simulink model "Scenario_3_PF"  (R2020b)
settings: Solver=ode1  StartTime=0.0  StopTime=10.0  RelTol=1e-3
InitFcn:
  | Scenario_3_parameters;
values from neighbouring files (symbols this model uses):
  c0 = c0_zeb    (= 6.57988e-09)    [Scenario_17_parameters_v2.m]    (also in Scenario_1_parameters_v2.m; Scenario_2_parameters_v2.m; Scenario_3_parameters_v2.m)
  c0_hawk = 6.37282e-09    [Scenario_17_parameters_v2.m]    (also in Scenario_1_parameters_v2.m; Scenario_2_parameters_v2.m; Scenario_3_parameters_v2.m)
  c1 = c1_zeb    (= 9.15905e-09)    [Scenario_17_parameters_v2.m]    (also in Scenario_1_parameters_v2.m; Scenario_2_parameters_v2.m; Scenario_3_parameters_v2.m)
  c1_hawk = 8.76156e-09    [Scenario_17_parameters_v2.m]    (also in Scenario_1_parameters_v2.m; Scenario_2_parameters_v2.m; Scenario_3_parameters_v2.m)
  fg = 50    [Scenario_17_parameters_v2.m]    (also in Scenario_1_parameters_v2.m; Scenario_2_parameters_v2.m; Scenario_3_parameters_v2.m)
  G10gen = 0.90    (= 0.9)    [Scenario_3_parameters_v2.m]
  G12gen = 0.85    [Scenario_3_parameters_v2.m]
  G1gen = 0.4692    [Scenario_17_parameters_v2.m]    (also in Scenario_1_parameters_v2.m = 0.1; Scenario_2_parameters_v2.m = 0.298581; Scenario_3_parameters_v2.m = 0.65)
  G2gen = 0.80    (= 0.8)    [Scenario_1_parameters_v2.m]    (also in Scenario_2_parameters_v2.m = 0.7; Scenario_3_parameters_v2.m = 0.4)
  G3gen = 0.85    [Scenario_1_parameters_v2.m]    (also in Scenario_2_parameters_v2.m = 0.9; Scenario_3_parameters_v2.m = 0.6)
  G4gen = 0.65    [Scenario_3_parameters_v2.m]
  G5gen = 0.75    [Scenario_17_parameters_v2.m]    (also in Scenario_1_parameters_v2.m = 0.8; Scenario_2_parameters_v2.m = 0.8; Scenario_3_parameters_v2.m = 0.705)
  G6gen = 0.90    (= 0.9)    [Scenario_17_parameters_v2.m]    (also in Scenario_1_parameters_v2.m; Scenario_2_parameters_v2.m = 0.81797; Scenario_3_parameters_v2.m = 0.45)
  G7gen = 0.20    (= 0.2)    [Scenario_17_parameters_v2.m]    (also in Scenario_1_parameters_v2.m = 0.5227; Scenario_2_parameters_v2.m = 0.5098; Scenario_3_parameters_v2.m = 0.4)
  G8gen = 0.58    [Scenario_17_parameters_v2.m]    (also in Scenario_3_parameters_v2.m = 0.65)
  G9gen = 0.8833    [Scenario_17_parameters_v2.m]    (also in Scenario_3_parameters_v2.m = 0.9)
  Ihvpk = Ihv*sqrt(2)    [Scenario_17_parameters_v2.m]    (also in Scenario_1_parameters_v2.m; Scenario_2_parameters_v2.m; Scenario_3_parameters_v2.m)
  l0 = l0_zeb    (= 0.00368)    [Scenario_17_parameters_v2.m]    (also in Scenario_1_parameters_v2.m; Scenario_2_parameters_v2.m; Scenario_3_parameters_v2.m)
  l0_hawk = 0.00373    [Scenario_17_parameters_v2.m]    (also in Scenario_1_parameters_v2.m; Scenario_2_parameters_v2.m; Scenario_3_parameters_v2.m)
  l1 = l1_zeb    (= 0.00128)    [Scenario_17_parameters_v2.m]    (also in Scenario_1_parameters_v2.m; Scenario_2_parameters_v2.m; Scenario_3_parameters_v2.m)
  L10dem = 0.04    [Scenario_3_parameters_v2.m]
  L12dem = 0.01    [Scenario_17_parameters_v2.m]    (also in Scenario_3_parameters_v2.m = 0.02)
  L13dem = 0.01    [Scenario_3_parameters_v2.m]
  l1_hawk = 0.00133    [Scenario_17_parameters_v2.m]    (also in Scenario_1_parameters_v2.m; Scenario_2_parameters_v2.m; Scenario_3_parameters_v2.m)
  L1dem = 0.25    [Scenario_17_parameters_v2.m]    (also in Scenario_3_parameters_v2.m = 0.1)
  L3dem = 0.30    (= 0.3)    [Scenario_17_parameters_v2.m]    (also in Scenario_1_parameters_v2.m = 0.1; Scenario_2_parameters_v2.m = 0.1; Scenario_3_parameters_v2.m = 0.2)
  L6dem = 0.15    [Scenario_1_parameters_v2.m]    (also in Scenario_2_parameters_v2.m; Scenario_3_parameters_v2.m = 0.1)
  L7dem = 0.10    (= 0.1)    [Scenario_1_parameters_v2.m]    (also in Scenario_2_parameters_v2.m; Scenario_3_parameters_v2.m = 0.2)
  L9dem = 0.15    [Scenario_17_parameters_v2.m]    (also in Scenario_3_parameters_v2.m = 0.1)
  Pr = Sr*PF    (= 1600500000)    [Scenario_17_parameters_v2.m]    (also in Scenario_1_parameters_v2.m = 1472500000; Scenario_2_parameters_v2.m = 1805000000; Scenario_3_parameters_v2.m = 12740000000)
  Qr = sqrt(Sr^2 - Pr^2)    [Scenario_17_parameters_v2.m]    (also in Scenario_1_parameters_v2.m; Scenario_2_parameters_v2.m; Scenario_3_parameters_v2.m)
  r0 = r0_zeb    (= 0.39362)    [Scenario_17_parameters_v2.m]    (also in Scenario_1_parameters_v2.m; Scenario_2_parameters_v2.m; Scenario_3_parameters_v2.m)
  r0_hawk = 0.44587    [Scenario_17_parameters_v2.m]    (also in Scenario_1_parameters_v2.m; Scenario_2_parameters_v2.m; Scenario_3_parameters_v2.m)
  r1 = r1_zeb    (= 0.06862)    [Scenario_17_parameters_v2.m]    (also in Scenario_1_parameters_v2.m; Scenario_2_parameters_v2.m; Scenario_3_parameters_v2.m)
  r1_hawk = 0.12087    [Scenario_17_parameters_v2.m]    (also in Scenario_1_parameters_v2.m; Scenario_2_parameters_v2.m; Scenario_3_parameters_v2.m)
  Rtpu = Xtpu/40    (= 0.0025)    [Scenario_17_parameters_v2.m]    (also in Scenario_1_parameters_v2.m = 0.00375; Scenario_2_parameters_v2.m = 0.00375; Scenario_3_parameters_v2.m)
  S10non = 500e6    (= 500000000)    [Scenario_3_parameters_v2.m]
  S12non = 250e6    (= 250000000)    [Scenario_3_parameters_v2.m]
  S1non = 700e6    (= 700000000)    [Scenario_17_parameters_v2.m]    (also in Scenario_1_parameters_v2.m = 400000000; Scenario_2_parameters_v2.m = 400000000; Scenario_3_parameters_v2.m = 1000000000)
  S2non = 300e6    (= 300000000)    [Scenario_1_parameters_v2.m]    (also in Scenario_2_parameters_v2.m; Scenario_3_parameters_v2.m = 3000000000)
  S3non = 200e6    (= 200000000)    [Scenario_1_parameters_v2.m]    (also in Scenario_2_parameters_v2.m; Scenario_3_parameters_v2.m = 1000000000)
  S4non = 2000e6    (= 2000000000)    [Scenario_3_parameters_v2.m]
  S5non = 400e6    (= 400000000)    [Scenario_17_parameters_v2.m]    (also in Scenario_1_parameters_v2.m = 500000000; Scenario_2_parameters_v2.m = 500000000; Scenario_3_parameters_v2.m = 2000000000)
  S6non = 150e6    (= 150000000)    [Scenario_17_parameters_v2.m]    (also in Scenario_1_parameters_v2.m = 400000000; Scenario_2_parameters_v2.m = 400000000; Scenario_3_parameters_v2.m = 3000000000)
  S7non = 1500e6    (= 1500000000)    [Scenario_17_parameters_v2.m]    (also in Scenario_1_parameters_v2.m = 200000000; Scenario_2_parameters_v2.m = 200000000; Scenario_3_parameters_v2.m = 4000000000)
  S8non = 600e6    (= 600000000)    [Scenario_17_parameters_v2.m]    (also in Scenario_3_parameters_v2.m = 2000000000)
  S9non = 200e6    (= 200000000)    [Scenario_17_parameters_v2.m]    (also in Scenario_3_parameters_v2.m = 1500000000)
  tonvsc = 0    [Scenario_17_parameters_v2.m]    (also in Scenario_1_parameters_v2.m; Scenario_2_parameters_v2.m; Scenario_3_parameters_v2.m = 0.0001)
  Ts = 50e-6    (= 5e-05)    [Scenario_17_parameters_v2.m]    (also in Scenario_1_parameters_v2.m = 0.0002; Scenario_2_parameters_v2.m = 2e-05; Scenario_3_parameters_v2.m = 0.0001)
  Vhv = 220e3    (= 220000)    [Scenario_17_parameters_v2.m]    (also in Scenario_1_parameters_v2.m; Scenario_2_parameters_v2.m; Scenario_3_parameters_v2.m)
  Vmv = 22e3    (= 22000)    [Scenario_17_parameters_v2.m]    (also in Scenario_1_parameters_v2.m; Scenario_2_parameters_v2.m; Scenario_3_parameters_v2.m)
  wc1 = wsw1/10    (= 848.230016469)    [Scenario_17_parameters_v2.m]    (also in Scenario_1_parameters_v2.m; Scenario_2_parameters_v2.m; Scenario_3_parameters_v2.m)
  wdc1 = wc1/10    (= 84.8230016469)    [Scenario_17_parameters_v2.m]    (also in Scenario_1_parameters_v2.m; Scenario_2_parameters_v2.m; Scenario_3_parameters_v2.m)
  wpq1 = wc1/10    (= 84.8230016469)    [Scenario_17_parameters_v2.m]    (also in Scenario_1_parameters_v2.m; Scenario_2_parameters_v2.m; Scenario_3_parameters_v2.m)
  wsw1 = ksw1*2*pi*fg    (= 8482.30016469)    [Scenario_17_parameters_v2.m]    (also in Scenario_1_parameters_v2.m; Scenario_2_parameters_v2.m; Scenario_3_parameters_v2.m)
  Xtpu = 0.10    (= 0.1)    [Scenario_17_parameters_v2.m]    (also in Scenario_1_parameters_v2.m = 0.15; Scenario_2_parameters_v2.m = 0.15; Scenario_3_parameters_v2.m)
undefined symbols (not defined in the file or in its folder): D11, Delta, Kf, r, theta0
libraries: powerlib x426, simulink_extras x305, powerlib_meascontrol x139, pid_lib x109, eeGeneralControl x72, simulink x60, eeTransforms x54, spsFirstOrderFilterLib x36, eePwmGeneratorTwoLevel x9
(part 5 of 36)

== system Scenario_3_PF/G9 ==
  Bus Selector : BusSelector  OutputSignals=Pabc,Qabc,f
  VSC : Subsystem  mask{vscmod=Phasor I-ref, fg=fg, Vhv=Vmv, Vmv=Vmv, Pconv=S9non, Rtpu=Rtpu, Xtpu=Xtpu, Hvsc=30e-3, qmode=Active power, dmode=Reactive power, wsw=wsw1, wn_pll=2*pi*80, wc=wc1, wpq=wpq1, wdc=wdc1, koc=1.2, tfilt=1*(1/wsw1), negseq_en=off, fdroop_en=on, Vacdroop_en=on, LVRT_en=off, Kfdroop=0.05, Kvdroop=0.1, Vlvrt0=0.9, Vlvrt_min=0.5, Qmax_lvrt=0.9}
      mask prompts: vscmod "VSC Model"; fg "AC grid frequency (Hz)"; Vhv "Grid-side voltage (V)(LL-rms)"; Vmv "Converter-side voltage (V)(LL-rms)"; Pconv "Converter nominal power (VA)"; Rtpu "Resistance seen by the converter (p.u)"; Xtpu "Reactance seen by the converter (p.u)"; Hvsc "VSC equivalent inertia (s)"; qmode "q-axis control mode"; dmode "d-axis control mode"; wsw "Switching frequency (rad/s)"; wn_pll "PLL filter natural frequency"; wc "Current-control bandwidth (rad/s)"; wpq "PQ control bandwidth (rad/s)"; wdc "DC Voltage control bandwidth(rad/s)"; koc "Overcurrent factor (p.u)"; tfilt "Vabc filter time constant (s)"; negseq_en "Enable negative sequence control"; fdroop_en "Enable frequency droop"; Vacdroop_en "Enable AC voltage droop"; LVRT_en "Enable LVRT"; Kfdroop "Frequency droop (p.u)"; Kvdroop "Voltage droop (p.u)"; Vlvrt0 "initial voltage (p.u)"; Vlvrt_min "minimum voltage (p.u)"; Qmax_lvrt "max power injected at min voltage (p.u)"
      mask init: same as Scenario_3_PF/G1/VSC
      mask TypeOptions vscmod: EMT Switching | EMT Average | Phasor Quasi-EMT | Phasor I-1st | Phasor I-ref | Phasor PQ-1st
      mask Callback vscmod:
      | % Control parameter visiblity
      | 
      | % Get the value of the Enable Bias checkbox
      | % unchecked = 'off'
      | % checked = 'on'
      | 
      | maskObj = Simulink.Mask.get(gcb);
      | 
      | wn_pll = 'on';
      | wsw = 'on';
      | vscmod = get_param(gcb,'vscmod');
      |     if strcmp(vscmod,'EMT Switching')
      |       wn_pll = 'on';
      |       wsw = 'on';
      |       tfilt = 'on';
      |     elseif strcmp(vscmod,'EMT Average')
      |         wn_pll = 'on';
      |         wsw = 'off';
      |         tfilt = 'off';
      |     elseif strcmp(vscmod,'Phasor Quasi-EMT')
      |         wn_pll = 'off';
      |         wsw = 'off';
      |         tfilt = 'off';
      |     elseif strcmp(vscmod,'Phasor I-1st')
      |         wn_pll = 'off';
      |         wsw = 'off';
      |         tfilt = 'off';
      |     elseif strcmp(vscmod,'Phasor I-ref')
      |         wn_pll = 'off';
      |         wsw = 'off';
      |         tfilt = 'off';
      |     elseif strcmp(vscmod,'Phasor PQ-1st')
      |         wn_pll = 'off';
      |         wsw = 'off';
      |         tfilt = 'off';
      |     end
      | 
      | fdroop_en = get_param(gcb,'fdroop_en');
      | Vacdroop_en = get_param(gcb,'Vacdroop_en');
      | LVRT_en = get_param(gcb,'LVRT_en');
      | negseq_en = get_param(gcb,'negseq_en');
      | 
      | % Set the 'MaskVisibilities' property for each parameters
      |     set_param(gcb,'MaskVisibilities',{'on','on','on','on','on','on','on','on','on','on',wsw,wn_pll,'on','on','on','on',tfilt,'on','on','on','on',fdroop_en,Vacdroop_en,'on','on','on'});
      | 
      | % Make LVRT area visible when it is enabled
      | if strcmp(LVRT_en,'on')
      |   maskObj.getDialogControl('Container_LVRT').Visible = 'on';
      | else
      |     maskObj.getDialogControl('Container_LVRT').Visible = 'off';
      | end
      | 
      | % Note that the value of the bias is not handled here.
      | % See the Initialization tab
      mask TypeOptions qmode: Active power | DC voltage
      mask Callback qmode:
      | %if strcmp(qmode,'Active Power')
      | %    disp(qmode)
      | %elseif strcmp(qmode,'DC Voltage')
      | %    disp(qmode)
      | %end
      mask TypeOptions dmode: Reactive power | AC voltage
      mask Callback fdroop_en:
      | % Control parameter visiblity
      | 
      | % Get the value of the Enable Bias checkbox
      | % unchecked = 'off'
      | % checked = 'on'
      | 
      | maskObj = Simulink.Mask.get(gcb);
      | 
      | wn_pll = 'on';
      | wsw = 'on';
      | vscmod = get_param(gcb,'vscmod');
      |     if strcmp(vscmod,'EMT Switching')
      |       wn_pll = 'on';
      |       wsw = 'on';
      |       tfilt = 'on';
      |     elseif strcmp(vscmod,'EMT Average')
      |         wn_pll = 'on';
      |         wsw = 'off';
      |         tfilt = 'off';
      |     elseif strcmp(vscmod,'Phasor Quasi-EMT')
      |         wn_pll = 'off';
      |         wsw = 'off';
      |         tfilt = 'off';
      |     elseif strcmp(vscmod,'Phasor I-1st')
      |         wn_pll = 'off';
      |         wsw = 'off';
      |         tfilt = 'off';
      |     elseif strcmp(vscmod,'Phasor I-ref')
      |         wn_pll = 'off';
      |         wsw = 'off';
      |         tfilt = 'off';
      |     elseif strcmp(vscmod,'Phasor PQ-1st')
      |         wn_pll = 'off';
      |         wsw = 'off';
      |         tfilt = 'off';
      |     end
      | 
      | fdroop_en = get_param(gcb,'fdroop_en');
      | Vacdroop_en = get_param(gcb,'Vacdroop_en');
      | LVRT_en = get_param(gcb,'LVRT_en');
      | negseq_en = get_param(gcb,'negseq_en');
      | 
      | % Set the 'MaskVisibilities' property for each parameters
      |     set_param(gcb,'MaskVisibilities',{'on','on','on','on','on','on','on','on','on','on',wsw,wn_pll,'on','on','on','on',tfilt,'on','on','on','on',fdroop_en,Vacdroop_en,'on','on','on'});
      | 
      | % Make LVRT area visible when it is enabled
      | if strcmp(LVRT_en,'on')
      |   maskObj.getDialogControl('Container_LVRT').Visible = 'on';
      | else
      |     maskObj.getDialogControl('Container_LVRT').Visible = 'off';
      | end
      | 
      | % Note that the value of the bias is not handled here.
      | % See the Initialization tab
      mask Callback Vacdroop_en:
      | % Control parameter visiblity
      | 
      | % Get the value of the Enable Bias checkbox
      | % unchecked = 'off'
      | % checked = 'on'
      | 
      | maskObj = Simulink.Mask.get(gcb);
      | 
      | wn_pll = 'on';
      | wsw = 'on';
      | vscmod = get_param(gcb,'vscmod');
      |     if strcmp(vscmod,'EMT Switching')
      |       wn_pll = 'on';
      |       wsw = 'on';
      |       tfilt = 'on';
      |     elseif strcmp(vscmod,'EMT Average')
      |         wn_pll = 'on';
      |         wsw = 'off';
      |         tfilt = 'off';
      |     elseif strcmp(vscmod,'Phasor Quasi-EMT')
      |         wn_pll = 'off';
      |         wsw = 'off';
      |         tfilt = 'off';
      |     elseif strcmp(vscmod,'Phasor I-1st')
      |         wn_pll = 'off';
      |         wsw = 'off';
      |         tfilt = 'off';
      |     elseif strcmp(vscmod,'Phasor I-ref')
      |         wn_pll = 'off';
      |         wsw = 'off';
      |         tfilt = 'off';
      |     elseif strcmp(vscmod,'Phasor PQ-1st')
      |         wn_pll = 'off';
      |         wsw = 'off';
      |         tfilt = 'off';
      |     end
      | 
      | fdroop_en = get_param(gcb,'fdroop_en');
      | Vacdroop_en = get_param(gcb,'Vacdroop_en');
      | LVRT_en = get_param(gcb,'LVRT_en');
      | negseq_en = get_param(gcb,'negseq_en');
      | 
      | % Set the 'MaskVisibilities' property for each parameters
      |     set_param(gcb,'MaskVisibilities',{'on','on','on','on','on','on','on','on','on','on',wsw,wn_pll,'on','on','on','on',tfilt,'on','on','on','on',fdroop_en,Vacdroop_en,'on','on','on'});
      | 
      | % Make LVRT area visible when it is enabled
      | if strcmp(LVRT_en,'on')
      |   maskObj.getDialogControl('Container_LVRT').Visible = 'on';
      | else
      |     maskObj.getDialogControl('Container_LVRT').Visible = 'off';
      | end
      | 
      | % Note that the value of the bias is not handled here.
      | % See the Initialization tab
      mask Callback LVRT_en:
      | % Control parameter visiblity
      | 
      | % Get the value of the Enable Bias checkbox
      | % unchecked = 'off'
      | % checked = 'on'
      | 
      | maskObj = Simulink.Mask.get(gcb);
      | 
      | wn_pll = 'on';
      | wsw = 'on';
      | vscmod = get_param(gcb,'vscmod');
      |     if strcmp(vscmod,'EMT Switching')
      |       wn_pll = 'on';
      |       wsw = 'on';
      |       tfilt = 'on';
      |     elseif strcmp(vscmod,'EMT Average')
      |         wn_pll = 'on';
      |         wsw = 'off';
      |         tfilt = 'off';
      |     elseif strcmp(vscmod,'Phasor Quasi-EMT')
      |         wn_pll = 'off';
      |         wsw = 'off';
      |         tfilt = 'off';
      |     elseif strcmp(vscmod,'Phasor I-1st')
      |         wn_pll = 'off';
      |         wsw = 'off';
      |         tfilt = 'off';
      |     elseif strcmp(vscmod,'Phasor I-ref')
      |         wn_pll = 'off';
      |         wsw = 'off';
      |         tfilt = 'off';
      |     elseif strcmp(vscmod,'Phasor PQ-1st')
      |         wn_pll = 'off';
      |         wsw = 'off';
      |         tfilt = 'off';
      |     end
      | 
      | fdroop_en = get_param(gcb,'fdroop_en');
      | Vacdroop_en = get_param(gcb,'Vacdroop_en');
      | LVRT_en = get_param(gcb,'LVRT_en');
      | negseq_en = get_param(gcb,'negseq_en');
      | 
      | % Set the 'MaskVisibilities' property for each parameters
      |     set_param(gcb,'MaskVisibilities',{'on','on','on','on','on','on','on','on','on','on',wsw,wn_pll,'on','on','on','on',tfilt,'on','on','on','on',fdroop_en,Vacdroop_en,'on','on','on'});
      | 
      | % Make LVRT area visible when it is enabled
      | if strcmp(LVRT_en,'on')
      |   maskObj.getDialogControl('Container_LVRT').Visible = 'on';
      | else
      |     maskObj.getDialogControl('Container_LVRT').Visible = 'off';
      | end
      | 
      | % Note that the value of the bias is not handled here.
      | % See the Initialization tab
      mask DialogControl DescTextVar Prompt: Three-phase VSC model
      mask DialogControl Tab1 Prompt: Electrical parameters
      mask DialogControl Tab2 Prompt: Control parameters
      mask DialogControl Tab3 Prompt: Other parameters
      mask DialogControl Container_LVRT Prompt: LVRT
      mask Display:
      | choice = get_param(gcb,'vscmod');
      | if strcmp(choice,'Phasor Quasi-EMT')
      |     disp('VSC\n\n')
      |     disp('\n\nPhasor\n\n')
      |     disp('\n\nQuasi-EMT')
      | elseif strcmp(choice,'EMT Average')
      |     disp('VSC\n')
      |     disp('\nEMT AVG')
      | elseif strcmp(choice,'EMT Switching')
      |     disp('VSC\n')
      |     disp('\nEMT SW')
      | elseif strcmp(choice,'Phasor I-1st')
      |     disp('VSC\n\n')
      |     disp('\n\nPhasor\n\n')
      |     disp('\n\nI 1st')
      | elseif strcmp(choice,'Phasor I-ref')
      |     disp('VSC\n\n')
      |     disp('\n\nPhasor\n\n')
      |     disp('\n\nI ref')
      | elseif strcmp(choice,'Phasor PQ-1st')
      |     disp('VSC\n\n')
      |     disp('\n\nPhasor\n\n')
      |     disp('\n\nPQ 1st')
      | end
  A : PMIOPort  Side=Right
  B : PMIOPort  Port=2  Side=Right
  C : PMIOPort  Port=3  Side=Right
  tag scope: Pg9=global, Qg9=global, fg9=global
  wires:
  VSC/1(m) -> Bus Selector/1
  Bus Selector/2 -> [Qg9]  "<Qabc>"
  Bus Selector/1 -> [Pg9]  "<Pabc>"
  Bus Selector/3 -> [fg9]  "<f>"
  connections:
  VSC/LConn2 -- B/RConn1
  VSC/LConn1 -- A/RConn1
  VSC/LConn3 -- C/RConn1

== system Scenario_3_PF/HVDC interconnection ==
  note: DC Link dynamics
  note: avoid division by zero
  Bus Selector1 : BusSelector  OutputSignals=Pabc,Qabc
  Bus Selector2 : BusSelector  OutputSignals=Pabc,Qabc,f
  Divide : Product  Inputs=*/
  Divide1 : Product  Inputs=*/
  Pset1 : Step  Time=3*tonvsc  After=-S8non*G8gen  SampleTime=0
  Qset1 : Step  Time=tonvsc  After=-30e6  SampleTime=0
  Qset2 : Step  Time=3*tonvsc  After=-400e6  SampleTime=0
  Saturation : Saturate  UpperLimit=10*Vhv  LowerLimit=1
  Saturation1 : Saturate  UpperLimit=10*Vhv  LowerLimit=1
  Subsystem1 : Subsystem  mask{C1=3100e-6/2, C2=3100e-6/2, R=5, L=100e-3, Vdc0=2*Vhv*sqrt(2)/sqrt(3)}
      mask prompts: C1 "Terminal 1 capacitance (F)"; C2 "Termina 2 capacitance (F)"; R "Link series resistance (Ohm)"; L "Link series inductance (H)"; Vdc0 "Link Initial voltage (V)"
      mask Display:
      | disp('back-to-back\n')
      | disp('\nDC link')
  Unit Delay : UnitDelay  SampleTime=-1  HasFrameUpgradeWarning=on
  Unit Delay1 : UnitDelay  SampleTime=-1  HasFrameUpgradeWarning=on
  VSC1 : Subsystem  mask{vscmod=Phasor I-ref, fg=fg, Vhv=Vhv, Vmv=Vhv, Pconv=S8non, Rtpu=Rtpu, Xtpu=Xtpu, Hvsc=30e-3, qmode=Active power, dmode=Reactive power, wsw=wsw1, wn_pll=2*pi*80, wc=wc1, wpq=wpq1, wdc=wdc1, koc=1.2, tfilt=1*(1/wsw1), negseq_en=off, fdroop_en=off, Vacdroop_en=off, LVRT_en=off, Kfdroop=0.05, Kvdroop=0.1, Vlvrt0=0.9, Vlvrt_min=0.5, Qmax_lvrt=0.9}
      mask prompts: vscmod "VSC Model"; fg "AC grid frequency (Hz)"; Vhv "Grid-side voltage (V)(LL-rms)"; Vmv "Converter-side voltage (V)(LL-rms)"; Pconv "Converter nominal power (VA)"; Rtpu "Resistance seen by the converter (p.u)"; Xtpu "Reactance seen by the converter (p.u)"; Hvsc "VSC equivalent inertia (s)"; qmode "q-axis control mode"; dmode "d-axis control mode"; wsw "Switching frequency (rad/s)"; wn_pll "PLL filter natural frequency"; wc "Current-control bandwidth (rad/s)"; wpq "PQ control bandwidth (rad/s)"; wdc "DC Voltage control bandwidth(rad/s)"; koc "Overcurrent factor (p.u)"; tfilt "Vabc filter time constant (s)"; negseq_en "Enable negative sequence control"; fdroop_en "Enable frequency droop"; Vacdroop_en "Enable AC voltage droop"; LVRT_en "Enable LVRT"; Kfdroop "Frequency droop (p.u)"; Kvdroop "Voltage droop (p.u)"; Vlvrt0 "initial voltage (p.u)"; Vlvrt_min "minimum voltage (p.u)"; Qmax_lvrt "max power injected at min voltage (p.u)"
      mask init: same as Scenario_3_PF/G1/VSC
      mask TypeOptions vscmod: EMT Switching | EMT Average | Phasor Quasi-EMT | Phasor I-1st | Phasor I-ref | Phasor PQ-1st
      mask Callback vscmod:
      | % Control parameter visiblity
      | 
      | % Get the value of the Enable Bias checkbox
      | % unchecked = 'off'
      | % checked = 'on'
      | 
      | maskObj = Simulink.Mask.get(gcb);
      | 
      | wn_pll = 'on';
      | wsw = 'on';
      | vscmod = get_param(gcb,'vscmod');
      |     if strcmp(vscmod,'EMT Switching')
      |       wn_pll = 'on';
      |       wsw = 'on';
      |       tfilt = 'on';
      |     elseif strcmp(vscmod,'EMT Average')
      |         wn_pll = 'on';
      |         wsw = 'off';
      |         tfilt = 'off';
      |     elseif strcmp(vscmod,'Phasor Quasi-EMT')
      |         wn_pll = 'off';
      |         wsw = 'off';
      |         tfilt = 'off';
      |     elseif strcmp(vscmod,'Phasor I-1st')
      |         wn_pll = 'off';
      |         wsw = 'off';
      |         tfilt = 'off';
      |     elseif strcmp(vscmod,'Phasor I-ref')
      |         wn_pll = 'off';
      |         wsw = 'off';
      |         tfilt = 'off';
      |     elseif strcmp(vscmod,'Phasor PQ-1st')
      |         wn_pll = 'off';
      |         wsw = 'off';
      |         tfilt = 'off';
      |     end
      | 
      | fdroop_en = get_param(gcb,'fdroop_en');
      | Vacdroop_en = get_param(gcb,'Vacdroop_en');
      | LVRT_en = get_param(gcb,'LVRT_en');
      | negseq_en = get_param(gcb,'negseq_en');
      | 
      | % Set the 'MaskVisibilities' property for each parameters
      |     set_param(gcb,'MaskVisibilities',{'on','on','on','on','on','on','on','on','on','on',wsw,wn_pll,'on','on','on','on',tfilt,'on','on','on','on',fdroop_en,Vacdroop_en,'on','on','on'});
      | 
      | % Make LVRT area visible when it is enabled
      | if strcmp(LVRT_en,'on')
      |   maskObj.getDialogControl('Container_LVRT').Visible = 'on';
      | else
      |     maskObj.getDialogControl('Container_LVRT').Visible = 'off';
      | end
      | 
      | % Note that the value of the bias is not handled here.
      | % See the Initialization tab
      mask TypeOptions qmode: Active power | DC voltage
      mask Callback qmode:
      | %if strcmp(qmode,'Active Power')
      | %    disp(qmode)
      | %elseif strcmp(qmode,'DC Voltage')
      | %    disp(qmode)
      | %end
      mask TypeOptions dmode: Reactive power | AC voltage
      mask Callback fdroop_en:
      | % Control parameter visiblity
      | 
      | % Get the value of the Enable Bias checkbox
      | % unchecked = 'off'
      | % checked = 'on'
      | 
      | maskObj = Simulink.Mask.get(gcb);
      | 
      | wn_pll = 'on';
      | wsw = 'on';
      | vscmod = get_param(gcb,'vscmod');
      |     if strcmp(vscmod,'EMT Switching')
      |       wn_pll = 'on';
      |       wsw = 'on';
      |       tfilt = 'on';
      |     elseif strcmp(vscmod,'EMT Average')
      |         wn_pll = 'on';
      |         wsw = 'off';
      |         tfilt = 'off';
      |     elseif strcmp(vscmod,'Phasor Quasi-EMT')
      |         wn_pll = 'off';
      |         wsw = 'off';
      |         tfilt = 'off';
      |     elseif strcmp(vscmod,'Phasor I-1st')
      |         wn_pll = 'off';
      |         wsw = 'off';
      |         tfilt = 'off';
      |     elseif strcmp(vscmod,'Phasor I-ref')
      |         wn_pll = 'off';
      |         wsw = 'off';
      |         tfilt = 'off';
      |     elseif strcmp(vscmod,'Phasor PQ-1st')
      |         wn_pll = 'off';
      |         wsw = 'off';
      |         tfilt = 'off';
      |     end
      | 
      | fdroop_en = get_param(gcb,'fdroop_en');
      | Vacdroop_en = get_param(gcb,'Vacdroop_en');
      | LVRT_en = get_param(gcb,'LVRT_en');
      | negseq_en = get_param(gcb,'negseq_en');
      | 
      | % Set the 'MaskVisibilities' property for each parameters
      |     set_param(gcb,'MaskVisibilities',{'on','on','on','on','on','on','on','on','on','on',wsw,wn_pll,'on','on','on','on',tfilt,'on','on','on','on',fdroop_en,Vacdroop_en,'on','on','on'});
      | 
      | % Make LVRT area visible when it is enabled
      | if strcmp(LVRT_en,'on')
      |   maskObj.getDialogControl('Container_LVRT').Visible = 'on';
      | else
      |     maskObj.getDialogControl('Container_LVRT').Visible = 'off';
      | end
      | 
      | % Note that the value of the bias is not handled here.
      | % See the Initialization tab
      mask Callback Vacdroop_en:
      | % Control parameter visiblity
      | 
      | % Get the value of the Enable Bias checkbox
      | % unchecked = 'off'
      | % checked = 'on'
      | 
      | maskObj = Simulink.Mask.get(gcb);
      | 
      | wn_pll = 'on';
      | wsw = 'on';
      | vscmod = get_param(gcb,'vscmod');
      |     if strcmp(vscmod,'EMT Switching')
      |       wn_pll = 'on';
      |       wsw = 'on';
      |       tfilt = 'on';
      |     elseif strcmp(vscmod,'EMT Average')
      |         wn_pll = 'on';
      |         wsw = 'off';
      |         tfilt = 'off';
      |     elseif strcmp(vscmod,'Phasor Quasi-EMT')
      |         wn_pll = 'off';
      |         wsw = 'off';
      |         tfilt = 'off';
      |     elseif strcmp(vscmod,'Phasor I-1st')
      |         wn_pll = 'off';
      |         wsw = 'off';
      |         tfilt = 'off';
      |     elseif strcmp(vscmod,'Phasor I-ref')
      |         wn_pll = 'off';
      |         wsw = 'off';
      |         tfilt = 'off';
      |     elseif strcmp(vscmod,'Phasor PQ-1st')
      |         wn_pll = 'off';
      |         wsw = 'off';
      |         tfilt = 'off';
      |     end
      | 
      | fdroop_en = get_param(gcb,'fdroop_en');
      | Vacdroop_en = get_param(gcb,'Vacdroop_en');
      | LVRT_en = get_param(gcb,'LVRT_en');
      | negseq_en = get_param(gcb,'negseq_en');
      | 
      | % Set the 'MaskVisibilities' property for each parameters
      |     set_param(gcb,'MaskVisibilities',{'on','on','on','on','on','on','on','on','on','on',wsw,wn_pll,'on','on','on','on',tfilt,'on','on','on','on',fdroop_en,Vacdroop_en,'on','on','on'});
      | 
      | % Make LVRT area visible when it is enabled
      | if strcmp(LVRT_en,'on')
      |   maskObj.getDialogControl('Container_LVRT').Visible = 'on';
      | else
      |     maskObj.getDialogControl('Container_LVRT').Visible = 'off';
      | end
      | 
      | % Note that the value of the bias is not handled here.
      | % See the Initialization tab
      mask Callback LVRT_en:
      | % Control parameter visiblity
      | 
      | % Get the value of the Enable Bias checkbox
      | % unchecked = 'off'
      | % checked = 'on'
      | 
      | maskObj = Simulink.Mask.get(gcb);
      | 
      | wn_pll = 'on';
      | wsw = 'on';
      | vscmod = get_param(gcb,'vscmod');
      |     if strcmp(vscmod,'EMT Switching')
      |       wn_pll = 'on';
      |       wsw = 'on';
      |       tfilt = 'on';
      |     elseif strcmp(vscmod,'EMT Average')
      |         wn_pll = 'on';
      |         wsw = 'off';
      |         tfilt = 'off';
      |     elseif strcmp(vscmod,'Phasor Quasi-EMT')
      |         wn_pll = 'off';
      |         wsw = 'off';
      |         tfilt = 'off';
      |     elseif strcmp(vscmod,'Phasor I-1st')
      |         wn_pll = 'off';
      |         wsw = 'off';
      |         tfilt = 'off';
      |     elseif strcmp(vscmod,'Phasor I-ref')
      |         wn_pll = 'off';
      |         wsw = 'off';
      |         tfilt = 'off';
      |     elseif strcmp(vscmod,'Phasor PQ-1st')
      |         wn_pll = 'off';
      |         wsw = 'off';
      |         tfilt = 'off';
      |     end
      | 
      | fdroop_en = get_param(gcb,'fdroop_en');
      | Vacdroop_en = get_param(gcb,'Vacdroop_en');
      | LVRT_en = get_param(gcb,'LVRT_en');
      | negseq_en = get_param(gcb,'negseq_en');
      | 
      | % Set the 'MaskVisibilities' property for each parameters
      |     set_param(gcb,'MaskVisibilities',{'on','on','on','on','on','on','on','on','on','on',wsw,wn_pll,'on','on','on','on',tfilt,'on','on','on','on',fdroop_en,Vacdroop_en,'on','on','on'});
      | 
      | % Make LVRT area visible when it is enabled
      | if strcmp(LVRT_en,'on')
      |   maskObj.getDialogControl('Container_LVRT').Visible = 'on';
      | else
      |     maskObj.getDialogControl('Container_LVRT').Visible = 'off';
      | end
      | 
      | % Note that the value of the bias is not handled here.
      | % See the Initialization tab
      mask DialogControl DescTextVar Prompt: Three-phase VSC model
      mask DialogControl Tab1 Prompt: Electrical parameters
      mask DialogControl Tab2 Prompt: Control parameters
      mask DialogControl Tab3 Prompt: Other parameters
      mask DialogControl Container_LVRT Prompt: LVRT
      mask Display:
      | choice = get_param(gcb,'vscmod');
      | if strcmp(choice,'Phasor Quasi-EMT')
      |     disp('VSC\n\n')
      |     disp('\n\nPhasor\n\n')
      |     disp('\n\nQuasi-EMT')
      | elseif strcmp(choice,'EMT Average')
      |     disp('VSC\n')
      |     disp('\nEMT AVG')
      | elseif strcmp(choice,'EMT Switching')
      |     disp('VSC\n')
      |     disp('\nEMT SW')
      | elseif strcmp(choice,'Phasor I-1st')
      |     disp('VSC\n\n')
      |     disp('\n\nPhasor\n\n')
      |     disp('\n\nI 1st')
      | elseif strcmp(choice,'Phasor I-ref')
      |     disp('VSC\n\n')
      |     disp('\n\nPhasor\n\n')
      |     disp('\n\nI ref')
      | elseif strcmp(choice,'Phasor PQ-1st')
      |     disp('VSC\n\n')
      |     disp('\n\nPhasor\n\n')
      |     disp('\n\nPQ 1st')
      | end
  VSC2 : Subsystem  mask{vscmod=Phasor I-ref, fg=fg, Vhv=Vhv, Vmv=Vhv, Pconv=S8non, Rtpu=Rtpu, Xtpu=Xtpu, Hvsc=100e-3, qmode=DC voltage, dmode=Reactive power, wsw=wsw1, wn_pll=2*pi*80, wc=wc1, wpq=wpq1, wdc=wdc1, koc=1.2, tfilt=1*(1/wsw1), negseq_en=off, fdroop_en=off, Vacdroop_en=off, LVRT_en=off, Kfdroop=0.05, Kvdroop=0.1, Vlvrt0=0.9, Vlvrt_min=0.5, Qmax_lvrt=0.9}
      mask prompts: vscmod "VSC Model"; fg "AC grid frequency (Hz)"; Vhv "Grid-side voltage (V)(LL-rms)"; Vmv "Converter-side voltage (V)(LL-rms)"; Pconv "Converter nominal power (VA)"; Rtpu "Resistance seen by the converter (p.u)"; Xtpu "Reactance seen by the converter (p.u)"; Hvsc "VSC equivalent inertia (s)"; qmode "q-axis control mode"; dmode "d-axis control mode"; wsw "Switching frequency (rad/s)"; wn_pll "PLL filter natural frequency"; wc "Current-control bandwidth (rad/s)"; wpq "PQ control bandwidth (rad/s)"; wdc "DC Voltage control bandwidth(rad/s)"; koc "Overcurrent factor (p.u)"; tfilt "Vabc filter time constant (s)"; negseq_en "Enable negative sequence control"; fdroop_en "Enable frequency droop"; Vacdroop_en "Enable AC voltage droop"; LVRT_en "Enable LVRT"; Kfdroop "Frequency droop (p.u)"; Kvdroop "Voltage droop (p.u)"; Vlvrt0 "initial voltage (p.u)"; Vlvrt_min "minimum voltage (p.u)"; Qmax_lvrt "max power injected at min voltage (p.u)"
      mask init: same as Scenario_3_PF/G1/VSC
      mask TypeOptions vscmod: EMT Switching | EMT Average | Phasor Quasi-EMT | Phasor I-1st | Phasor I-ref | Phasor PQ-1st
      mask Callback vscmod:
      | % Control parameter visiblity
      | 
      | % Get the value of the Enable Bias checkbox
      | % unchecked = 'off'
      | % checked = 'on'
      | 
      | maskObj = Simulink.Mask.get(gcb);
      | 
      | wn_pll = 'on';
      | wsw = 'on';
      | vscmod = get_param(gcb,'vscmod');
      |     if strcmp(vscmod,'EMT Switching')
      |       wn_pll = 'on';
      |       wsw = 'on';
      |       tfilt = 'on';
      |     elseif strcmp(vscmod,'EMT Average')
      |         wn_pll = 'on';
      |         wsw = 'off';
      |         tfilt = 'off';
      |     elseif strcmp(vscmod,'Phasor Quasi-EMT')
      |         wn_pll = 'off';
      |         wsw = 'off';
      |         tfilt = 'off';
      |     elseif strcmp(vscmod,'Phasor I-1st')
      |         wn_pll = 'off';
      |         wsw = 'off';
      |         tfilt = 'off';
      |     elseif strcmp(vscmod,'Phasor I-ref')
      |         wn_pll = 'off';
      |         wsw = 'off';
      |         tfilt = 'off';
      |     elseif strcmp(vscmod,'Phasor PQ-1st')
      |         wn_pll = 'off';
      |         wsw = 'off';
      |         tfilt = 'off';
      |     end
      | 
      | fdroop_en = get_param(gcb,'fdroop_en');
      | Vacdroop_en = get_param(gcb,'Vacdroop_en');
      | LVRT_en = get_param(gcb,'LVRT_en');
      | negseq_en = get_param(gcb,'negseq_en');
      | 
      | % Set the 'MaskVisibilities' property for each parameters
      |     set_param(gcb,'MaskVisibilities',{'on','on','on','on','on','on','on','on','on','on',wsw,wn_pll,'on','on','on','on',tfilt,'on','on','on','on',fdroop_en,Vacdroop_en,'on','on','on'});
      | 
      | % Make LVRT area visible when it is enabled
      | if strcmp(LVRT_en,'on')
      |   maskObj.getDialogControl('Container_LVRT').Visible = 'on';
      | else
      |     maskObj.getDialogControl('Container_LVRT').Visible = 'off';
      | end
      | 
      | % Note that the value of the bias is not handled here.
      | % See the Initialization tab
      mask TypeOptions qmode: Active power | DC voltage
      mask Callback qmode:
      | %if strcmp(qmode,'Active Power')
      | %    disp(qmode)
      | %elseif strcmp(qmode,'DC Voltage')
      | %    disp(qmode)
      | %end
      mask TypeOptions dmode: Reactive power | AC voltage
      mask Callback fdroop_en:
      | % Control parameter visiblity
      | 
      | % Get the value of the Enable Bias checkbox
      | % unchecked = 'off'
      | % checked = 'on'
      | 
      | maskObj = Simulink.Mask.get(gcb);
      | 
      | wn_pll = 'on';
      | wsw = 'on';
      | vscmod = get_param(gcb,'vscmod');
      |     if strcmp(vscmod,'EMT Switching')
      |       wn_pll = 'on';
      |       wsw = 'on';
      |       tfilt = 'on';
      |     elseif strcmp(vscmod,'EMT Average')
      |         wn_pll = 'on';
      |         wsw = 'off';
      |         tfilt = 'off';
      |     elseif strcmp(vscmod,'Phasor Quasi-EMT')
      |         wn_pll = 'off';
      |         wsw = 'off';
      |         tfilt = 'off';
      |     elseif strcmp(vscmod,'Phasor I-1st')
      |         wn_pll = 'off';
      |         wsw = 'off';
      |         tfilt = 'off';
      |     elseif strcmp(vscmod,'Phasor I-ref')
      |         wn_pll = 'off';
      |         wsw = 'off';
      |         tfilt = 'off';
      |     elseif strcmp(vscmod,'Phasor PQ-1st')
      |         wn_pll = 'off';
      |         wsw = 'off';
      |         tfilt = 'off';
      |     end
      | 
      | fdroop_en = get_param(gcb,'fdroop_en');
      | Vacdroop_en = get_param(gcb,'Vacdroop_en');
      | LVRT_en = get_param(gcb,'LVRT_en');
      | negseq_en = get_param(gcb,'negseq_en');
      | 
      | % Set the 'MaskVisibilities' property for each parameters
      |     set_param(gcb,'MaskVisibilities',{'on','on','on','on','on','on','on','on','on','on',wsw,wn_pll,'on','on','on','on',tfilt,'on','on','on','on',fdroop_en,Vacdroop_en,'on','on','on'});
      | 
      | % Make LVRT area visible when it is enabled
      | if strcmp(LVRT_en,'on')
      |   maskObj.getDialogControl('Container_LVRT').Visible = 'on';
      | else
      |     maskObj.getDialogControl('Container_LVRT').Visible = 'off';
      | end
      | 
      | % Note that the value of the bias is not handled here.
      | % See the Initialization tab
      mask Callback Vacdroop_en:
      | % Control parameter visiblity
      | 
      | % Get the value of the Enable Bias checkbox
      | % unchecked = 'off'
      | % checked = 'on'
      | 
      | maskObj = Simulink.Mask.get(gcb);
      | 
      | wn_pll = 'on';
      | wsw = 'on';
      | vscmod = get_param(gcb,'vscmod');
      |     if strcmp(vscmod,'EMT Switching')
      |       wn_pll = 'on';
      |       wsw = 'on';
      |       tfilt = 'on';
      |     elseif strcmp(vscmod,'EMT Average')
      |         wn_pll = 'on';
      |         wsw = 'off';
      |         tfilt = 'off';
      |     elseif strcmp(vscmod,'Phasor Quasi-EMT')
      |         wn_pll = 'off';
      |         wsw = 'off';
      |         tfilt = 'off';
      |     elseif strcmp(vscmod,'Phasor I-1st')
      |         wn_pll = 'off';
      |         wsw = 'off';
      |         tfilt = 'off';
      |     elseif strcmp(vscmod,'Phasor I-ref')
      |         wn_pll = 'off';
      |         wsw = 'off';
      |         tfilt = 'off';
      |     elseif strcmp(vscmod,'Phasor PQ-1st')
      |         wn_pll = 'off';
      |         wsw = 'off';
      |         tfilt = 'off';
      |     end
      | 
      | fdroop_en = get_param(gcb,'fdroop_en');
      | Vacdroop_en = get_param(gcb,'Vacdroop_en');
      | LVRT_en = get_param(gcb,'LVRT_en');
      | negseq_en = get_param(gcb,'negseq_en');
      | 
      | % Set the 'MaskVisibilities' property for each parameters
      |     set_param(gcb,'MaskVisibilities',{'on','on','on','on','on','on','on','on','on','on',wsw,wn_pll,'on','on','on','on',tfilt,'on','on','on','on',fdroop_en,Vacdroop_en,'on','on','on'});
      | 
      | % Make LVRT area visible when it is enabled
      | if strcmp(LVRT_en,'on')
      |   maskObj.getDialogControl('Container_LVRT').Visible = 'on';
      | else
      |     maskObj.getDialogControl('Container_LVRT').Visible = 'off';
      | end
      | 
      | % Note that the value of the bias is not handled here.
      | % See the Initialization tab
      mask Callback LVRT_en:
      | % Control parameter visiblity
      | 
      | % Get the value of the Enable Bias checkbox
      | % unchecked = 'off'
      | % checked = 'on'
      | 
      | maskObj = Simulink.Mask.get(gcb);
      | 
      | wn_pll = 'on';
      | wsw = 'on';
      | vscmod = get_param(gcb,'vscmod');
      |     if strcmp(vscmod,'EMT Switching')
      |       wn_pll = 'on';
      |       wsw = 'on';
      |       tfilt = 'on';
      |     elseif strcmp(vscmod,'EMT Average')
      |         wn_pll = 'on';
      |         wsw = 'off';
      |         tfilt = 'off';
      |     elseif strcmp(vscmod,'Phasor Quasi-EMT')
      |         wn_pll = 'off';
      |         wsw = 'off';
      |         tfilt = 'off';
      |     elseif strcmp(vscmod,'Phasor I-1st')
      |         wn_pll = 'off';
      |         wsw = 'off';
      |         tfilt = 'off';
      |     elseif strcmp(vscmod,'Phasor I-ref')
      |         wn_pll = 'off';
      |         wsw = 'off';
      |         tfilt = 'off';
      |     elseif strcmp(vscmod,'Phasor PQ-1st')
      |         wn_pll = 'off';
      |         wsw = 'off';
      |         tfilt = 'off';
      |     end
      | 
      | fdroop_en = get_param(gcb,'fdroop_en');
      | Vacdroop_en = get_param(gcb,'Vacdroop_en');
      | LVRT_en = get_param(gcb,'LVRT_en');
      | negseq_en = get_param(gcb,'negseq_en');
      | 
      | % Set the 'MaskVisibilities' property for each parameters
      |     set_param(gcb,'MaskVisibilities',{'on','on','on','on','on','on','on','on','on','on',wsw,wn_pll,'on','on','on','on',tfilt,'on','on','on','on',fdroop_en,Vacdroop_en,'on','on','on'});
      | 
      | % Make LVRT area visible when it is enabled
      | if strcmp(LVRT_en,'on')
      |   maskObj.getDialogControl('Container_LVRT').Visible = 'on';
      | else
      |     maskObj.getDialogControl('Container_LVRT').Visible = 'off';
      | end
      | 
      | % Note that the value of the bias is not handled here.
      | % See the Initialization tab
      mask DialogControl DescTextVar Prompt: Three-phase VSC model
      mask DialogControl Tab1 Prompt: Electrical parameters
      mask DialogControl Tab2 Prompt: Control parameters
      mask DialogControl Tab3 Prompt: Other parameters
      mask DialogControl Container_LVRT Prompt: LVRT
      mask Display:
      | choice = get_param(gcb,'vscmod');
      | if strcmp(choice,'Phasor Quasi-EMT')
      |     disp('VSC\n\n')
      |     disp('\n\nPhasor\n\n')
      |     disp('\n\nQuasi-EMT')
      | elseif strcmp(choice,'EMT Average')
      |     disp('VSC\n')
      |     disp('\nEMT AVG')
      | elseif strcmp(choice,'EMT Switching')
      |     disp('VSC\n')
      |     disp('\nEMT SW')
      | elseif strcmp(choice,'Phasor I-1st')
      |     disp('VSC\n\n')
      |     disp('\n\nPhasor\n\n')
      |     disp('\n\nI 1st')
      | elseif strcmp(choice,'Phasor I-ref')
      |     disp('VSC\n\n')
      |     disp('\n\nPhasor\n\n')
      |     disp('\n\nI ref')
      | elseif strcmp(choice,'Phasor PQ-1st')
      |     disp('VSC\n\n')
      |     disp('\n\nPhasor\n\n')
      |     disp('\n\nPQ 1st')
      | end
  A1 : PMIOPort  Side=Right
  B1 : PMIOPort  Port=2  Side=Right
  C1 : PMIOPort  Port=3  Side=Right
  A2 : PMIOPort  Port=4  Side=Left
  B2 : PMIOPort  Port=5  Side=Left
  C2 : PMIOPort  Port=6  Side=Left
  tag scope: Pac2=global, Pg8=global, Qac2=global, Qg8=global, fg8=global
  wires:
  Pset1/1 -> VSC1/1(Pset)
  Qset1/1 -> VSC1/2(Qset)
  [Pac1] -> Divide/1
  Divide/1 -> [idc1]
  [vdc1] -> Divide/2
  VSC1/1(m) -> Bus Selector2/1
  Qset2/1 -> VSC2/2(Qset)
  Bus Selector1/2 -> [Qac2]  "<Qabc>"
  Bus Selector1/1 -> [Pac2]  "<Pabc>"
  VSC2/1(m) -> Bus Selector1/1
  [vdc2] -> Divide1/2
  [Pac2] -> Divide1/1
  [vdc2] -> VSC2/3(Edc)
  [idc1] -> Unit Delay/1
  Unit Delay/1 -> Subsystem1/1(idc1)
  Unit Delay1/1 -> Subsystem1/2(idc2)
  [idc2] -> Unit Delay1/1
  Divide1/1 -> [idc2]
  Saturation/1 -> [vdc1]
  Saturation1/1 -> [vdc2]
  Subsystem1/1(vdc1) -> Saturation/1
  Subsystem1/2(vdc2) -> Saturation1/1
  Bus Selector2/2 -> [Qg8], [Qac1]  "<Qabc>"
  Bus Selector2/1 -> [Pg8], [Pac1]  "<Pabc>"
  Bus Selector2/3 -> [fg8]  "<f>"
  connections:
  VSC1/LConn2 -- B1/RConn1
  VSC1/LConn3 -- C1/RConn1
  A2/RConn1 -- VSC2/LConn1
  B2/RConn1 -- VSC2/LConn2
  C2/RConn1 -- VSC2/LConn3
  A1/RConn1 -- VSC1/LConn1

== system Scenario_3_PF/Measurements EMT ==
  Active power : Scope
  Frequency (Hz) : Scope
  Gain5 : Gain  Gain=fg
  Gain6 : Gain  Gain=fg
  Gain7 : Gain  Gain=fg
  Mux2 : Mux  Inputs=11
  Mux4 : Mux  Inputs=11
  Mux6 : Mux  Inputs=13
  "Power (3ph, Instantaneous)" : powerlib_meascontrol/Measurements/Power (3ph, Instantaneous)
  "Power (3ph, Instantaneous)1" : powerlib_meascontrol/Measurements/Power (3ph, Instantaneous)
  "Power (3ph, Instantaneous)2" : powerlib_meascontrol/Measurements/Power (3ph, Instantaneous)
  RMS{14..19,21..27} (13 alike) : powerlib_meascontrol/Measurements/RMS  TrueRMS=on  Freq=fg  RMSInit=0  Ts=0
  Scope2 : Scope
  tag scope: Pg2=global, Pg3=global, Pg5=global, Qg2=global, Qg3=global, Qg5=global
  wires:
  [I5] -> "Power (3ph, Instantaneous)2"/2
  [V5] -> "Power (3ph, Instantaneous)2"/1
  "Power (3ph, Instantaneous)2"/1 -> [Pg5]
  "Power (3ph, Instantaneous)2"/2 -> [Qg5]
  [V3] -> "Power (3ph, Instantaneous)1"/1
  "Power (3ph, Instantaneous)1"/2 -> [Qg3]
  "Power (3ph, Instantaneous)1"/1 -> [Pg3]
  [Ig3] -> "Power (3ph, Instantaneous)1"/2
  "Power (3ph, Instantaneous)"/2 -> [Qg2]
  "Power (3ph, Instantaneous)"/1 -> [Pg2]
  [I2] -> "Power (3ph, Instantaneous)"/2
  [V2] -> "Power (3ph, Instantaneous)"/1
  Mux6/1 -> Scope2/1
  RMS25/1 -> Mux6/11  "V11"
  [V5] -> RMS18/1
  [V9] -> RMS23/1
  [V7] -> RMS21/1
  [V13] -> RMS27/1
  [V8] -> RMS22/1
  [V6] -> RMS19/1
  [V3] -> RMS16/1
  [V11] -> RMS25/1
  RMS14/1 -> Mux6/1  "V1"
  RMS23/1 -> Mux6/9  "V9"
  RMS17/1 -> Mux6/4  "V4"
  RMS16/1 -> Mux6/3  "V3"
  RMS19/1 -> Mux6/6  "V6"
  RMS15/1 -> Mux6/2  "V2"
  RMS18/1 -> Mux6/5  "V5"
  [V10] -> RMS24/1
  [V1] -> RMS14/1
  [V4] -> RMS17/1
  RMS27/1 -> Mux6/13  "V13"
  [V12] -> RMS26/1
  RMS22/1 -> Mux6/8  "V8"
  RMS21/1 -> Mux6/7  "V7"
  RMS24/1 -> Mux6/10  "V10"
  RMS26/1 -> Mux6/12  "V12"
  [V2] -> RMS15/1
  [wm3] -> Gain6/1
  [wm2] -> Gain5/1
  Mux4/1 -> Frequency (Hz)/1
  [fg1] -> Mux4/1  "fg1"
  [wm5] -> Gain7/1
  [fg8] -> Mux4/8  "fg8"
  [fg7] -> Mux4/7  "fg7"
  [fg12] -> Mux4/11  "fg12"
  Gain7/1 -> Mux4/5  "fg5"
  [fg9] -> Mux4/9  "fg9"
  [fg10] -> Mux4/10  "fg10"
  [fg4] -> Mux4/4  "fg4"
  Gain6/1 -> Mux4/3  "fg3"
  Gain5/1 -> Mux4/2  "fg2"
  [fg6] -> Mux4/6  "fg6"
  [Pg10] -> Mux2/10  "Pg10"
  [Pg10] -> Mux2/11  "Pg12"
  [Pg4] -> Mux2/4  "Pg4"
  [Pg1] -> Mux2/1  "Pg1"
  [Pg8] -> Mux2/8  "Pg8"
  [Pg7] -> Mux2/7  "Pg7"
  Mux2/1 -> Active power/1
  [Pg3] -> Mux2/3  "Pg3"
  [Pg9] -> Mux2/9  "Pg9"
  [Pg2] -> Mux2/2  "Pg2"
  [Pg5] -> Mux2/5  "Pg5"
  [Pg6] -> Mux2/6  "Pg6"
